simulink model "Diagrama_blocos"  (R2021a)
settings: Solver=VariableStepAuto  StartTime=0.0  StopTime=10.0  RelTol=1e-3
libraries: visiontextngfix x6
settings Model: Creator=V  LastModifiedBy=V

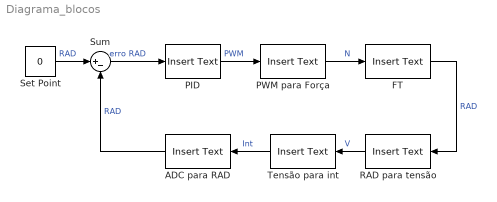
== system Diagrama_blocos ==
  ADC para RAD : visiontextngfix/Insert Text  inputType=Obsolete  theText=H2  getTextLocFrom=Specify via dialog  textLoc=[1 1]  getTextColorFrom=Specify via dialog  textColor=[0 0 0]  getTextIntensityFrom=Specify via dialog  textIntensity=0  getTextOpacityFrom=Specify via dialog  textOpacity=1.0  dummyVar2=0  dummyVar3=0  dummyVar4=0  imagePorts=One multidimensional signal  isInputTransposed=off  fontFace=LucidaSansRegular  dummyVar1=0  blockFontSize=12  antiAliased=on
      settings: SourceProductBaseCode=VP
  FT : visiontextngfix/Insert Text  inputType=Obsolete  theText=G  getTextLocFrom=Specify via dialog  textLoc=[1 1]  getTextColorFrom=Specify via dialog  textColor=[0 0 0]  getTextIntensityFrom=Specify via dialog  textIntensity=0  getTextOpacityFrom=Specify via dialog  textOpacity=1.0  dummyVar2=0  dummyVar3=0  dummyVar4=0  imagePorts=One multidimensional signal  isInputTransposed=off  fontFace=LucidaSansRegular  dummyVar1=0  blockFontSize=12  antiAliased=on
      settings: SourceProductBaseCode=VP
  PID : visiontextngfix/Insert Text  inputType=Obsolete  theText=PID  getTextLocFrom=Specify via dialog  textLoc=[1 1]  getTextColorFrom=Specify via dialog  textColor=[0 0 0]  getTextIntensityFrom=Specify via dialog  textIntensity=0  getTextOpacityFrom=Specify via dialog  textOpacity=1.0  dummyVar2=0  dummyVar3=0  dummyVar4=0  imagePorts=One multidimensional signal  isInputTransposed=off  fontFace=LucidaSansRegular  dummyVar1=0  blockFontSize=12  antiAliased=on
      settings: SourceProductBaseCode=VP
  PWM para Força : visiontextngfix/Insert Text  inputType=Obsolete  theText=H1  getTextLocFrom=Specify via dialog  textLoc=[1 1]  getTextColorFrom=Specify via dialog  textColor=[0 0 0]  getTextIntensityFrom=Specify via dialog  textIntensity=0  getTextOpacityFrom=Specify via dialog  textOpacity=1.0  dummyVar2=0  dummyVar3=0  dummyVar4=0  imagePorts=One multidimensional signal  isInputTransposed=off  fontFace=LucidaSansRegular  dummyVar1=0  blockFontSize=12  antiAliased=on
      settings: SourceProductBaseCode=VP
  RAD para tensão : visiontextngfix/Insert Text  inputType=Obsolete  theText=Sensor  getTextLocFrom=Specify via dialog  textLoc=[1 1]  getTextColorFrom=Specify via dialog  textColor=[0 0 0]  getTextIntensityFrom=Specify via dialog  textIntensity=0  getTextOpacityFrom=Specify via dialog  textOpacity=1.0  dummyVar2=0  dummyVar3=0  dummyVar4=0  imagePorts=One multidimensional signal  isInputTransposed=off  fontFace=LucidaSansRegular  dummyVar1=0  blockFontSize=12  antiAliased=on
      settings: SourceProductBaseCode=VP
  Set Point : Constant  Value=0
  Sum : Sum  Inputs=|+-
  Tensão para int : visiontextngfix/Insert Text  inputType=Obsolete  theText=ADC  getTextLocFrom=Specify via dialog  textLoc=[1 1]  getTextColorFrom=Specify via dialog  textColor=[0 0 0]  getTextIntensityFrom=Specify via dialog  textIntensity=0  getTextOpacityFrom=Specify via dialog  textOpacity=1.0  dummyVar2=0  dummyVar3=0  dummyVar4=0  imagePorts=One multidimensional signal  isInputTransposed=off  fontFace=LucidaSansRegular  dummyVar1=0  blockFontSize=12  antiAliased=on
      settings: SourceProductBaseCode=VP
  wires:
  PID/1 -> PWM para Força/1  "PWM"
  PWM para Força/1 -> FT/1  "N"
  Tensão para int/1 -> ADC para RAD/1  "Int"
  ADC para RAD/1 -> Sum/2  "RAD"
  Sum/1 -> PID/1  "erro RAD"
  Set Point/1 -> Sum/1  "RAD"
  RAD para tensão/1 -> Tensão para int/1  "V"
  FT/1 -> RAD para tensão/1  "RAD"
